simulink model "chap11_3sim"  (Simulink 7.7)
settings: Solver=ode45  StartTime=0.0  StopTime=10  FixedStep=0.001  RelTol=1e-3
settings Model: Creator=ljk  LastModifiedBy=ljk  ExtModeTrigMode=oneshot  ExtModeArmWhenConnect=off
settings DataIOCC: LimitDataPoints=off  SignalLoggingName=sigsOut
settings OptimizationCC: BooleanDataType=off
settings DebuggingCC: SaveWithParameterizedLinksMsg=none  SignalResolutionControl=TryResolveAllWithWarning  SolverPrmCheckMsg=none  MultiTaskDSMMsg=warning  MultiTaskCondExecSysMsg=none  StrictBusMsg=None
settings HardwareCC: TargetUnknown=on
settings RTWCC: IncludeERTFirstTime=on

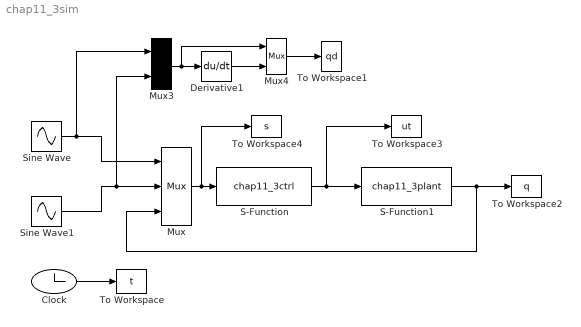
== system chap11_3sim ==
  Clock : Clock
  Derivative1 : Derivative
  Mux : Mux  Inputs=3
  Mux3 : Mux  Inputs=2
  Mux4 : Mux  Inputs=2
  S-Function : S-Function  FunctionName=chap11_3ctrl  EnableBusSupport=off
  S-Function1 : S-Function  FunctionName=chap11_3plant  EnableBusSupport=off
  Sine Wave : Sin  Phase=pi/2  SampleTime=0
  Sine Wave1 : Sin  SampleTime=0
  To Workspace : ToWorkspace  VariableName=t  SampleTime=-1  SaveFormat=Array
  To Workspace1 : ToWorkspace  VariableName=qd  SampleTime=-1  SaveFormat=Array
  To Workspace2 : ToWorkspace  VariableName=q  SampleTime=-1  SaveFormat=Array
  To Workspace3 : ToWorkspace  VariableName=ut  SampleTime=-1  SaveFormat=Array
  To Workspace4 : ToWorkspace  VariableName=s  SampleTime=-1  SaveFormat=Array
  wires:
  Mux/1 -> S-Function/1, To Workspace4/1
  Sine Wave/1 -> Mux/1, Mux3/1
  S-Function/1 -> S-Function1/1, To Workspace3/1
  Sine Wave1/1 -> Mux/2, Mux3/2
  S-Function1/1 -> Mux/3, To Workspace2/1
  Clock/1 -> To Workspace/1
  Derivative1/1 -> Mux4/2
  Mux3/1 -> Derivative1/1, Mux4/1
  Mux4/1 -> To Workspace1/1
